simulink model "Task2P"  (R2022a)
settings: Solver=FixedStepAuto  StartTime=0.0  StopTime=10  FixedStep=0.001  RelTol=1e-3
undefined symbols (not defined in the file): k_avg, kp1, kp2, kp3, Tm_avg, y
settings Model: Creator=Family  LastModifiedBy=Family

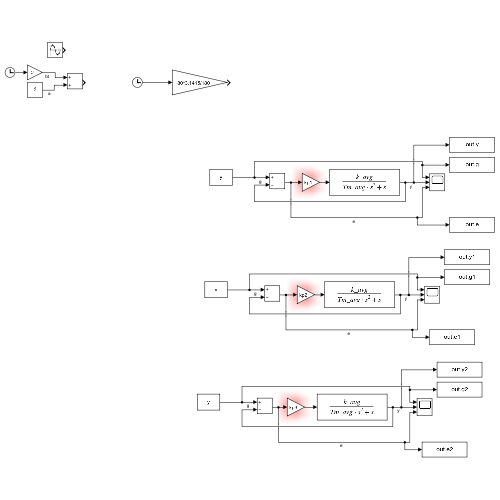
[thumbnail: Simulink's stored preview of the top-level diagram]
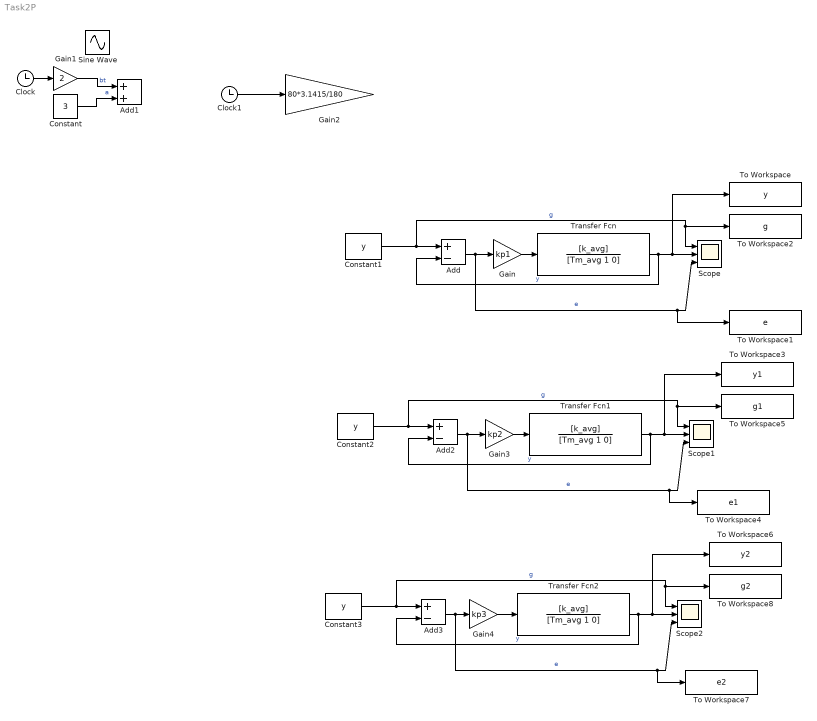
== system Task2P ==
  Add : Sum  Inputs=+-
  Add1 : Sum
  Add2 : Sum  Inputs=+-
  Add3 : Sum  Inputs=+-
  Clock : Clock
  Clock1 : Clock
  Constant : Constant  Value=3
  Constant1 : Constant  Value=y  SampleTime=-1
  Constant2 : Constant  Value=y  SampleTime=-1
  Constant3 : Constant  Value=y  SampleTime=-1
  Gain : Gain  Gain=kp1
  Gain1 : Gain  Gain=2
  Gain2 : Gain  Gain=80*3.1415/180
  Gain3 : Gain  Gain=kp2
  Gain4 : Gain  Gain=kp3
  Scope : Scope  NumInputPorts=3
  Scope1 : Scope  NumInputPorts=3
  Scope2 : Scope  NumInputPorts=3
  Sine Wave : Sin  Amplitude=2  Phase=2  SampleTime=0
  To Workspace : ToWorkspace  VariableName=y  SaveFormat=Timeseries  SampleTime=-1
  To Workspace1 : ToWorkspace  VariableName=e  SaveFormat=Timeseries  SampleTime=-1
  To Workspace2 : ToWorkspace  VariableName=g  SaveFormat=Timeseries  SampleTime=-1
  To Workspace3 : ToWorkspace  VariableName=y1  SaveFormat=Timeseries  SampleTime=-1
  To Workspace4 : ToWorkspace  VariableName=e1  SaveFormat=Timeseries  SampleTime=-1
  To Workspace5 : ToWorkspace  VariableName=g1  SaveFormat=Timeseries  SampleTime=-1
  To Workspace6 : ToWorkspace  VariableName=y2  SaveFormat=Timeseries  SampleTime=-1
  To Workspace7 : ToWorkspace  VariableName=e2  SaveFormat=Timeseries  SampleTime=-1
  To Workspace8 : ToWorkspace  VariableName=g2  SaveFormat=Timeseries  SampleTime=-1
  Transfer Fcn : TransferFcn  Numerator=[k_avg]  Denominator=[Tm_avg 1 0]
  Transfer Fcn1 : TransferFcn  Numerator=[k_avg]  Denominator=[Tm_avg 1 0]
  Transfer Fcn2 : TransferFcn  Numerator=[k_avg]  Denominator=[Tm_avg 1 0]
  wires:
  Transfer Fcn/1 -> To Workspace/1, Scope/2, Add/2  "y"
  Add/1 -> To Workspace1/1, Scope/3, Gain/1  "e"
  Constant1/1 -> To Workspace2/1, Scope/1, Add/1  "g"
  Gain/1 -> Transfer Fcn/1
  Clock/1 -> Gain1/1
  Gain1/1 -> Add1/1  "bt"
  Constant/1 -> Add1/2  "a"
  Clock1/1 -> Gain2/1
  Add2/1 -> To Workspace4/1, Scope1/3, Gain3/1  "e"
  Gain3/1 -> Transfer Fcn1/1
  Transfer Fcn1/1 -> To Workspace3/1, Scope1/2, Add2/2  "y"
  Constant2/1 -> To Workspace5/1, Scope1/1, Add2/1  "g"
  Add3/1 -> To Workspace7/1, Scope2/3, Gain4/1  "e"
  Gain4/1 -> Transfer Fcn2/1
  Transfer Fcn2/1 -> To Workspace6/1, Scope2/2, Add3/2  "y"
  Constant3/1 -> To Workspace8/1, Scope2/1, Add3/1  "g"
